simulink model "flightinput2R50parameterestworkingga"  (R2014b)
settings: Solver=ode45  StartTime=6  StopTime=30  RelTol=1e-3
values from neighbouring files (symbols this model uses):
  A = [-0.00831112375605  -0.312191336457; 0.106560419114  -0.651132188207]    [Day1.mat]    (also in ParamCheck.m = [Xu,0,0,0,0,-9.81,Xa,0,0,0,0,0,0; ParamGA.m = [Xu,0,0,0,0,-9.81,Xa,0,0,0,0,0,0; Success.mat = [-0.0348422585102  1.24263627919; -0.0150642561243  -0.28228; usingCoherence.m = [Xu,0,0,0,0,-9.81,Xa,0,0,0,0,0,0)
  B = [0.00211649834197 0.00424685617202]    [Day1.mat]    (also in ParamCheck.m = [0,0,0,0; ParamGA.m = [0,0,0,0; Success.mat = [2.7077267635 -0.620250606455]; usingCoherence.m = [0,0,0,0)
  C = [-4.48857112979 0.320159784813]    [Day1.mat]    (also in ParamCheck.m = [cpop(1,1),0,0,0,0,0,0,0,0,0,0,0,0; ParamGA.m = eye(13); Success.mat = [-0.596439704268 0.724317666886]; usingCoherence.m = eye(13))
undefined symbols (not defined in the file or in its folder): sigbuilder_block
settings Model: ExtModeTrigMode=oneshot  ExtModeArmWhenConnect=off  ExtModeAutoUpdateStatusClock=off  Creator=The MathWorks Inc.  LastModifiedBy=Navaneeth Krishnan B
settings DataIOCC: LimitDataPoints=off  SignalLoggingSaveFormat=ModelDataLogs
settings OptimizationCC: BlockReduction=off  BooleanDataType=off  InitFltsAndDblsToZero=on
settings DebuggingCC: SaveWithParameterizedLinksMsg=none  UnderspecifiedInitializationDetection=Classic  MergeDetectMultiDrivingBlocksExec=none  SignalResolutionControl=TryResolveAllWithWarning  SolverPrmCheckMsg=none  MultiTaskDSMMsg=warning  MultiTaskCondExecSysMsg=none  FcnCallInpInsideContextMsg=UseLocalSettings  StateNameClashWarn=warning
settings HardwareCC: TargetHWDeviceType=32-bit Generic  ProdEqTarget=off
settings RTWCC: IncludeERTFirstTime=on
settings GRTTargetCC: TargetFcnLib=ansi_tfl_tmw.mat  CombineOutputUpdateFcns=off  GRTInterface=on

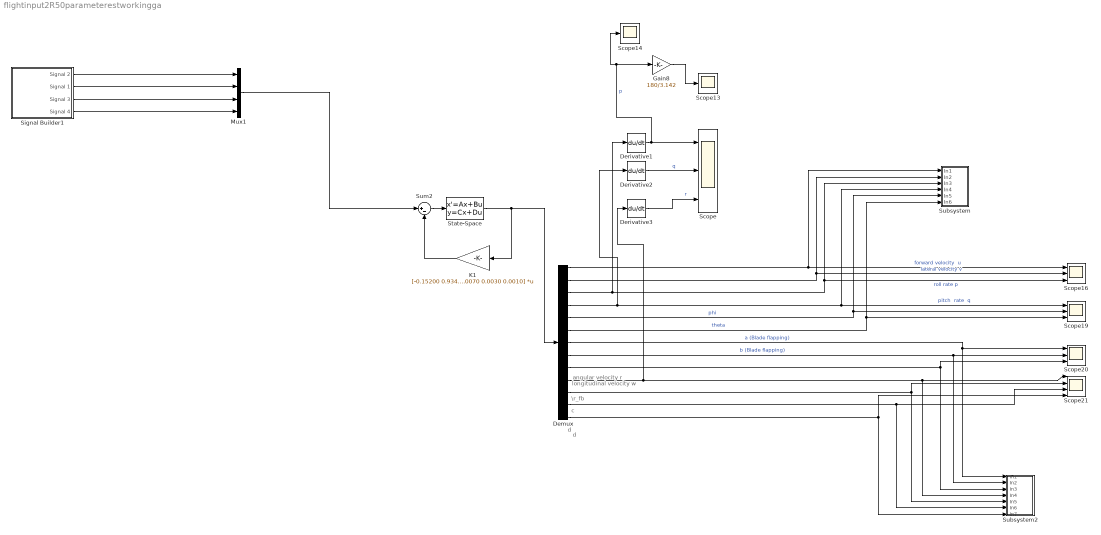
== system flightinput2R50parameterestworkingga ==
  note: d
  note: longitudinal velocity w
  note: d
  note: c
  note: \r_fb
  note: angular velocity r
  Demux : Demux  Outputs=13
  Derivative1 : Derivative
  Derivative2 : Derivative
  Derivative3 : Derivative
  Gain8 : Gain  Gain=180/3.142
  K1 : Gain  Gain="[-0.15200\t0.93400\t1.9290\t0.18900\t6.5360\t0.77700\t10.887\t66.050\t-0.0080\t0.074\t-0.12500\t-0.35200\t4.1590;0.97400\t0.14\t0.12200\t-2.5160\t0.74600\t-7.7990\t-64.275\t13.834\t-0.0020\t-0.051\t0.17100\t-3.9580\t0.29400;0.011\t-0.034\t-0.13400\t-0.013\t-0.21300\t-0.052\t-0.024\t-1.1640\t-0.023\t0.85400\t-0.53500\t0.010\t-0.0010;-0.0020\t-0.0070\t-0.018\t0.0040\t-0.047\t0.014\t0.28400\t2.2140\t-0.98600 -0.050\t0.0070\t0.0030\t0.0010]"  Multiplication=Matrix(K*u)  SaturateOnIntegerOverflow=on  OutDataTypeStr=Inherit: Same as input  ParamDataTypeStr=Inherit: Same as input
  Mux1 : Mux
  Scope{,16,19..20} (4 alike) : Scope  NumInputPorts=3
      Scope settings: TimeRange=10  YMin=-3e-05~-2e-06~-0.02  YMax=3e-05~2e-06~0.12  MaxDataPoints=5000000  SampleInput=on
      Scope16 settings: YMin=-5~-5~-5  YMax=5~5~5  SaveName=ScopeData16  MaxDataPoints=50000  SampleInput=on
      Scope19 settings: YMin=-5~-5~-5  YMax=5~5~5  SaveName=ScopeData19  MaxDataPoints=50000  SampleInput=on
      Scope20 settings: YMin=-5~-5~-5  YMax=5~5~5  SaveName=ScopeData20  MaxDataPoints=50000  SampleInput=on
  Scope13 : Scope
      settings: SaveName=ScopeData13  MaxDataPoints=50000  SampleInput=on
  Scope14 : Scope
      settings: SaveName=ScopeData14  MaxDataPoints=50000  SampleInput=on
  Scope21 : Scope  NumInputPorts=4
      settings: YMin=-5~-5~-5~-5  YMax=5~5~5~5  SaveName=ScopeData21  MaxDataPoints=50000  SampleInput=on
  Signal Builder1 : Subsystem  Tag=STV Subsys  LoadFcn=sigbuilder_block('load');  StartFcn=sigbuilder_block('start');  StopFcn=sigbuilder_block('stop');  ClipboardFcn=sigbuilder_block('clipboard');  mask(Sigbuilder block){}
      mask help: Simulink:masks:SigbuilderBlock_MD
      mask init:
      | if ~strcmp(get_param(bdroot(gcbh),'SimulationStatus'),'stopped') tuvar = sigbuilder_block('maskInit'); end
      settings: CopyFcn=sigbuilder_block('copy');  DeleteFcn=sigbuilder_block('delete');  ModelCloseFcn=sigbuilder_block('modelClose');  PreSaveFcn=sigbuilder_block('preSave');  PauseFcn=sigbuilder_block('pause');  ContinueFcn=sigbuilder_block('continue');  NameChangeFcn=sigbuilder_block('namechange');  OpenFcn=sigbuilder_block('open',[6 30.75 1012.5 481.5 ]);  CloseFcn=sigbuilder_block('close');
      mask Display: plot(0, 0, 100, 100,[2, 2, 32, 32, 2], [68, 8, 8, 68, 68],[32, 2], [38, 38], [32, 19, 2],[53, 60, 44], [32, 17, 17, 2],[16, 16, 31, 31]);txt = getActiveGroup(gcbh);text(2, 100, txt,'verticalAlignment', 'top');
  State-Space : StateSpace  A=A  B=B  C=C  D=zeros(8,2)  X0=0
  Subsystem : Subsystem
  Subsystem2 : Subsystem
  Sum2 : Sum  Inputs=|+-  SaturateOnIntegerOverflow=on  InputSameDT=on  OutDataTypeStr=Inherit: Same as first input
  wires:
  Demux/8 -> Scope20/2, Subsystem2/2(In2)  "b (Blade flapping)"
  Demux/7 -> Scope20/1, Subsystem2/1(In1)  "a (Blade flapping)"
  Demux/6 -> Scope19/3, Subsystem/6(In6)  "theta"
  Demux/5 -> Scope19/2, Subsystem/5(In5)  "phi"
  Demux/4 -> Derivative2/1, Scope19/1, Subsystem/4(In4)  "pitch  rate  q"
  Demux/3 -> Derivative1/1, Scope16/3, Subsystem/3(In3)  "roll rate p"
  Demux/2 -> Scope16/2, Subsystem/2(In2)  "lateral velocity v"
  Demux/1 -> Subsystem/1(In1), Scope16/1  "forward velocity  u"
  Demux/13 -> Scope21/4, Subsystem2/7(In7)
  Derivative1/1 -> Gain8/1, Scope14/1, Scope/1  "p"
  Derivative2/1 -> Scope/2  "q"
  Derivative3/1 -> Scope/3  "r"
  State-Space/1 -> K1/1, Demux/1
  K1/1 -> Sum2/2
  Sum2/1 -> State-Space/1
  Signal Builder1/1(Signal 2) -> Mux1/1
  Signal Builder1/2(Signal 1) -> Mux1/2
  Signal Builder1/3(Signal 3) -> Mux1/3
  Signal Builder1/4(Signal 4) -> Mux1/4
  Gain8/1 -> Scope13/1
  Demux/10 -> Derivative3/1, Scope21/1, Subsystem2/4(In4)
  Demux/11 -> Scope21/2, Subsystem2/5(In5)
  Demux/12 -> Scope21/3, Subsystem2/6(In6)
  Demux/9 -> Scope20/3, Subsystem2/3(In3)
  Mux1/1 -> Sum2/1

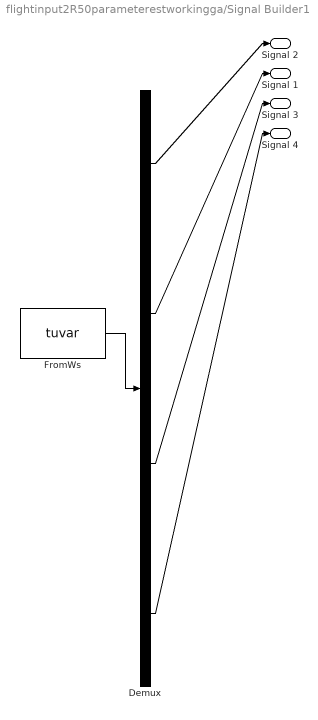
== system flightinput2R50parameterestworkingga/Signal Builder1 ==
  Demux : Demux  Tag=STV Demux
  FromWs : FromWorkspace  Tag=STV FromWs  VariableName=tuvar  SampleTime=0
      SigBuilderData=|
      | common.afterFinalStr = 'Extrapolate'
      | common.sampleTime = 0
      | dataSet.timeRange = [0 25]
      | dataSet.name = 'Group 1'
      | sbobj.Groups.Name = 'Group 1'
      | sbobj.Groups.Signals(1).Name = 'Signal 2'
      | sbobj.Groups.Signals(1).XData = [0 2.98 2.98 4 4 4.88 4.88 8 10 10 12 12 14 14 16 16 18 18 20 20 22 22 24 24 25]
      | sbobj.Groups.Signals(1).YData = [0 0 -0.02 0.28 -0.02 0.24 -0.26 -0.26 -0.26 -0.02 -0.02 0.22 0.22 0 0 -0.2 -0.2 0.14 0.14 0.16 0.16 -0.19 -0.19 0 0]
      | sbobj.Groups.Signals(2).Name = 'Signal 1'
      | sbobj.Groups.Signals(2).XData = [0 2 2 3.46 3.46 4.86 4.86 6.56 6.56 8.78 8.78 12 12 14 14 16 16 17.4 17.4 20 20 22 22 24 24 25]
      | sbobj.Groups.Signals(2).YData = [-0.02 -0.02 0.24 0.24 -0.24 -0.24 -0.02 -0.02 0.16 0.16 0.24 0.24 -0.12 -0.12 -0.21 -0.21 0.25 0.25 -0.18 -0.18 -0.09 -0.09 0.13 0.13 0 0]
      | sbobj.Groups.Signals(3).Name = 'Signal 3'
      | sbobj.Groups.Signals(3).XData = [0 2 4.56 4.56 4.78 4.78 5.7 5.7 6.8 6.8 7.36 7.36 8.82 8.82 9.3 9.3 9.76 9.76 12.72 12.72 13.52 13.52 24 25]
      | sbobj.Groups.Signals(3).YData = [0 0 0 0.32 0.32 -0.2 -0.2 0.22 0.22 -0.26 -0.26 0 0 -0.24 -0.24 0.34 0.34 0 0 0.2 0.2 0 0 0]
      | sbobj.Groups.Signals(4).Name = 'Signal 4'
      | sbobj.Groups.Signals(4).XData = [0 2 4 4 6 6 8 8 10 10 12 12 14 14 16 18 18 20 20 22 22 24 24 25]
      | sbobj.Groups.Signals(4).YData = [0 0 0 -0.08 -0.08 -0.26 -0.26 -0.16 -0.16 -0.26 -0.26 -0.1 -0.1 -0.24 -0.24 -0.24 -0.14 -0.14 -0.3 -0.3 -0.12 -0.12 -0.04 -0.04]
      | sbobj.Groups.TimeRange = [0 25]
  Signal 2 : Outport  Tag=STV Outport
  Signal 1 : Outport  Tag=STV Outport  Port=2
  Signal 3 : Outport  Tag=STV Outport  Port=3
  Signal 4 : Outport  Tag=STV Outport  Port=4
  wires:
  FromWs/1 -> Demux/1
  Demux/1 -> Signal 2/1
  Demux/2 -> Signal 1/1
  Demux/3 -> Signal 3/1
  Demux/4 -> Signal 4/1

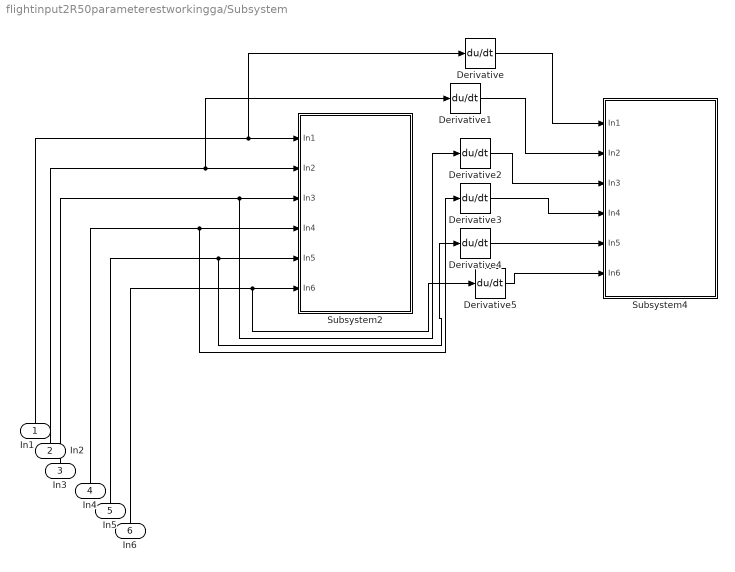
== system flightinput2R50parameterestworkingga/Subsystem ==
  In1 : Inport
  In2 : Inport  Port=2
  In3 : Inport  Port=3
  In4 : Inport  Port=4
  In5 : Inport  Port=5
  In6 : Inport  Port=6
  Derivative{,1..5} (6 alike) : Derivative
  Subsystem2 : Subsystem
  Subsystem4 : Subsystem
  wires:
  In6/1 -> Derivative5/1, Subsystem2/6(In6)
  In1/1 -> Derivative/1, Subsystem2/1(In1)
  In3/1 -> Derivative2/1, Subsystem2/3(In3)
  In5/1 -> Derivative4/1, Subsystem2/5(In5)
  In4/1 -> Derivative3/1, Subsystem2/4(In4)
  In2/1 -> Derivative1/1, Subsystem2/2(In2)
  Derivative2/1 -> Subsystem4/3(In3)
  Derivative1/1 -> Subsystem4/2(In2)
  Derivative3/1 -> Subsystem4/4(In4)
  Derivative4/1 -> Subsystem4/5(In5)
  Derivative/1 -> Subsystem4/1(In1)
  Derivative5/1 -> Subsystem4/6(In6)

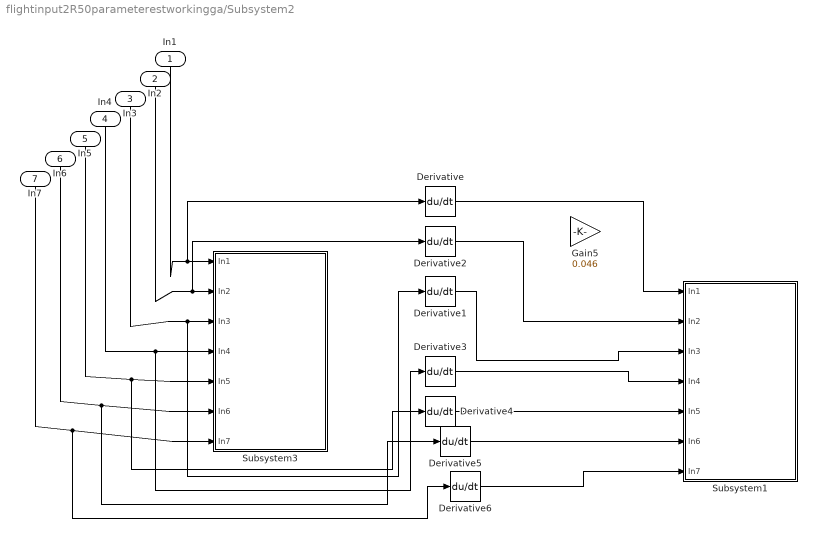
== system flightinput2R50parameterestworkingga/Subsystem2 ==
  In1 : Inport
  In2 : Inport  Port=2
  In3 : Inport  Port=3
  In4 : Inport  Port=4
  In5 : Inport  Port=5
  In6 : Inport  Port=6
  In7 : Inport  Port=7
  Derivative{,1..6} (7 alike) : Derivative
  Gain5 : Gain  Gain=0.046
  Subsystem1 : Subsystem
  Subsystem3 : Subsystem
  wires:
  In3/1 -> Derivative1/1, Subsystem3/3(In3)
  In4/1 -> Derivative3/1, Subsystem3/4(In4)
  In6/1 -> Derivative5/1, Subsystem3/6(In6)
  In7/1 -> Derivative6/1, Subsystem3/7(In7)
  In5/1 -> Derivative4/1, Subsystem3/5(In5)
  Derivative3/1 -> Subsystem1/4(In4)
  Derivative1/1 -> Subsystem1/3(In3)
  Derivative4/1 -> Subsystem1/5(In5)
  In1/1 -> Derivative/1, Subsystem3/1(In1)
  In2/1 -> Derivative2/1, Subsystem3/2(In2)
  Derivative5/1 -> Subsystem1/6(In6)
  Derivative/1 -> Subsystem1/1(In1)
  Derivative2/1 -> Subsystem1/2(In2)
  Derivative6/1 -> Subsystem1/7(In7)

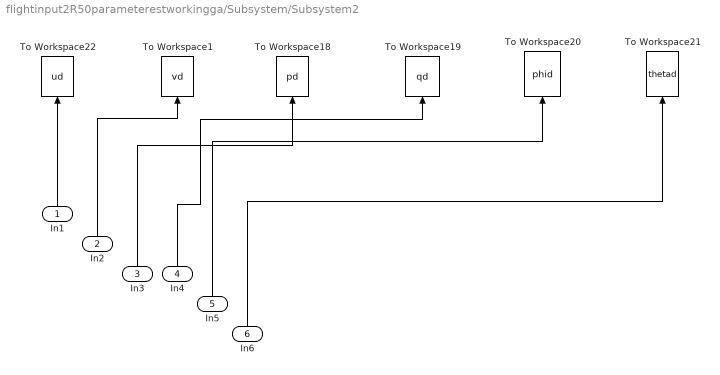
== system flightinput2R50parameterestworkingga/Subsystem/Subsystem2 ==
  In1 : Inport
  In2 : Inport  Port=2
  In3 : Inport  Port=3
  In4 : Inport  Port=4
  In5 : Inport  Port=5
  In6 : Inport  Port=6
  To Workspace1 : ToWorkspace  VariableName=vd  SampleTime=0.01
      settings: Save2DSignal=2-D array (concatenate along first dimension)
  To Workspace18 : ToWorkspace  VariableName=pd  SampleTime=0.01
      settings: Save2DSignal=2-D array (concatenate along first dimension)
  To Workspace19 : ToWorkspace  VariableName=qd  SampleTime=0.01
      settings: Save2DSignal=2-D array (concatenate along first dimension)
  To Workspace20 : ToWorkspace  VariableName=phid  SampleTime=0.01
      settings: Save2DSignal=2-D array (concatenate along first dimension)
  To Workspace21 : ToWorkspace  VariableName=thetad  SampleTime=0.01
  To Workspace22 : ToWorkspace  VariableName=ud  SampleTime=0.01
      settings: Save2DSignal=2-D array (concatenate along first dimension)
  wires:
  In1/1 -> To Workspace22/1
  In3/1 -> To Workspace18/1
  In4/1 -> To Workspace19/1
  In6/1 -> To Workspace21/1
  In5/1 -> To Workspace20/1
  In2/1 -> To Workspace1/1

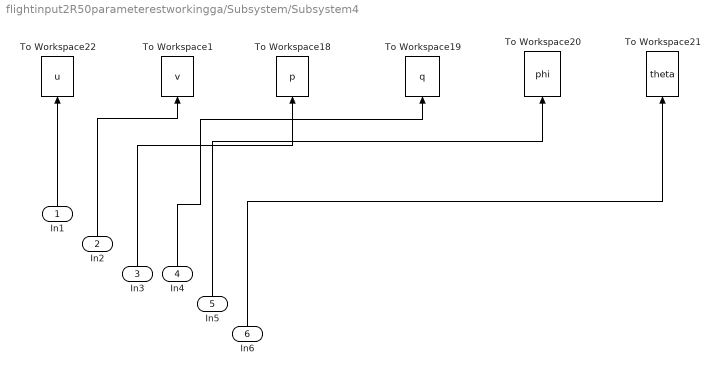
== system flightinput2R50parameterestworkingga/Subsystem/Subsystem4 ==
  In1 : Inport
  In2 : Inport  Port=2
  In3 : Inport  Port=3
  In4 : Inport  Port=4
  In5 : Inport  Port=5
  In6 : Inport  Port=6
  To Workspace1 : ToWorkspace  VariableName=v  SampleTime=0.01
      settings: Save2DSignal=2-D array (concatenate along first dimension)
  To Workspace18 : ToWorkspace  VariableName=p  SampleTime=0.01
      settings: Save2DSignal=2-D array (concatenate along first dimension)
  To Workspace19 : ToWorkspace  VariableName=q  SampleTime=0.01
      settings: Save2DSignal=2-D array (concatenate along first dimension)
  To Workspace20 : ToWorkspace  VariableName=phi  SampleTime=0.01
      settings: Save2DSignal=2-D array (concatenate along first dimension)
  To Workspace21 : ToWorkspace  VariableName=theta  SampleTime=0.01
  To Workspace22 : ToWorkspace  VariableName=u  SampleTime=0.01
      settings: Save2DSignal=2-D array (concatenate along first dimension)
  wires:
  In2/1 -> To Workspace1/1
  In5/1 -> To Workspace20/1
  In6/1 -> To Workspace21/1
  In4/1 -> To Workspace19/1
  In3/1 -> To Workspace18/1
  In1/1 -> To Workspace22/1

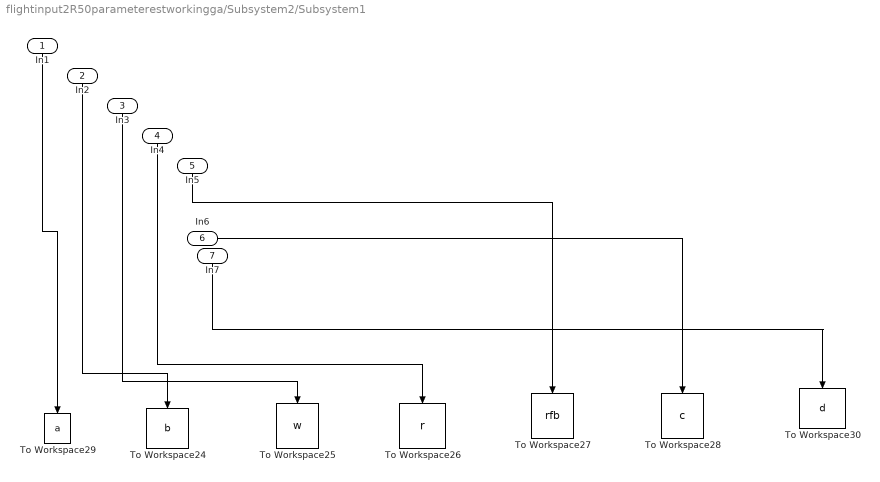
== system flightinput2R50parameterestworkingga/Subsystem2/Subsystem1 ==
  In1 : Inport
  In2 : Inport  Port=2
  In3 : Inport  Port=3
  In4 : Inport  Port=4
  In5 : Inport  Port=5
  In6 : Inport  Port=6
  In7 : Inport  Port=7
  To Workspace24 : ToWorkspace  VariableName=b  SampleTime=0.01
      settings: Save2DSignal=2-D array (concatenate along first dimension)
  To Workspace25 : ToWorkspace  VariableName=w  SampleTime=0.01
      settings: Save2DSignal=2-D array (concatenate along first dimension)
  To Workspace26 : ToWorkspace  VariableName=r  SampleTime=0.01
      settings: Save2DSignal=2-D array (concatenate along first dimension)
  To Workspace27 : ToWorkspace  VariableName=rfb  SampleTime=0.01
      settings: Save2DSignal=2-D array (concatenate along first dimension)
  To Workspace28 : ToWorkspace  VariableName=c  SampleTime=0.01
      settings: Save2DSignal=2-D array (concatenate along first dimension)
  To Workspace29 : ToWorkspace  VariableName=a  SampleTime=0.01
      settings: Save2DSignal=2-D array (concatenate along first dimension)
  To Workspace30 : ToWorkspace  VariableName=d  SampleTime=0.01
      settings: Save2DSignal=2-D array (concatenate along first dimension)
  wires:
  In6/1 -> To Workspace28/1
  In7/1 -> To Workspace30/1
  In2/1 -> To Workspace24/1
  In4/1 -> To Workspace26/1
  In3/1 -> To Workspace25/1
  In1/1 -> To Workspace29/1
  In5/1 -> To Workspace27/1

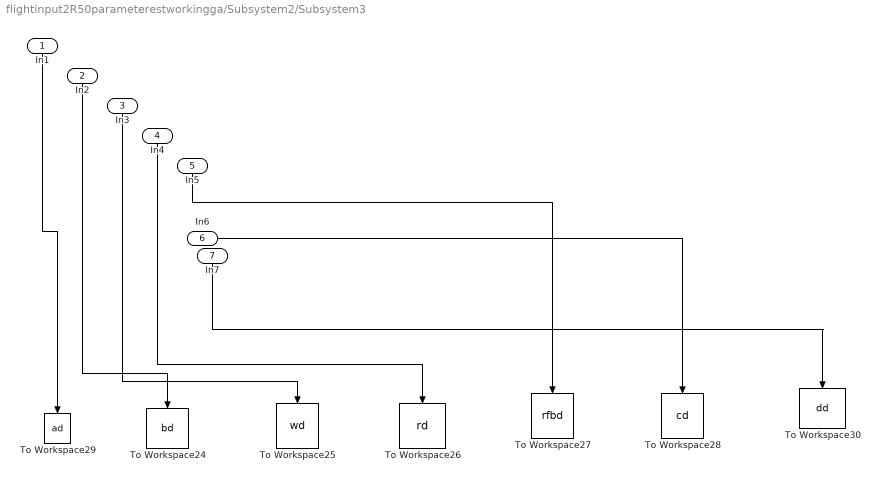
== system flightinput2R50parameterestworkingga/Subsystem2/Subsystem3 ==
  In1 : Inport
  In2 : Inport  Port=2
  In3 : Inport  Port=3
  In4 : Inport  Port=4
  In5 : Inport  Port=5
  In6 : Inport  Port=6
  In7 : Inport  Port=7
  To Workspace24 : ToWorkspace  VariableName=bd  SampleTime=0.01
      settings: Save2DSignal=2-D array (concatenate along first dimension)
  To Workspace25 : ToWorkspace  VariableName=wd  SampleTime=0.01
      settings: Save2DSignal=2-D array (concatenate along first dimension)
  To Workspace26 : ToWorkspace  VariableName=rd  SampleTime=0.01
      settings: Save2DSignal=2-D array (concatenate along first dimension)
  To Workspace27 : ToWorkspace  VariableName=rfbd  SampleTime=0.01
      settings: Save2DSignal=2-D array (concatenate along first dimension)
  To Workspace28 : ToWorkspace  VariableName=cd  SampleTime=0.01
      settings: Save2DSignal=2-D array (concatenate along first dimension)
  To Workspace29 : ToWorkspace  VariableName=ad  SampleTime=0.01
      settings: Save2DSignal=2-D array (concatenate along first dimension)
  To Workspace30 : ToWorkspace  VariableName=dd  SampleTime=0.01
      settings: Save2DSignal=2-D array (concatenate along first dimension)
  wires:
  In5/1 -> To Workspace27/1
  In1/1 -> To Workspace29/1
  In3/1 -> To Workspace25/1
  In4/1 -> To Workspace26/1
  In2/1 -> To Workspace24/1
  In7/1 -> To Workspace30/1
  In6/1 -> To Workspace28/1
